simulink model "signalTesting"  (R2024b)
settings: Solver=VariableStepAuto  StartTime=0.0  StopTime=60  RelTol=1e-3
libraries: dspstat3 x12, dspfdesign x6
settings Model: Creator=Mateusz  LastModifiedBy=Mateusz
settings OptimizationCC: ReuseModelBlockBuffer=off
settings RTWCC: GPUComputeCapability=3.5

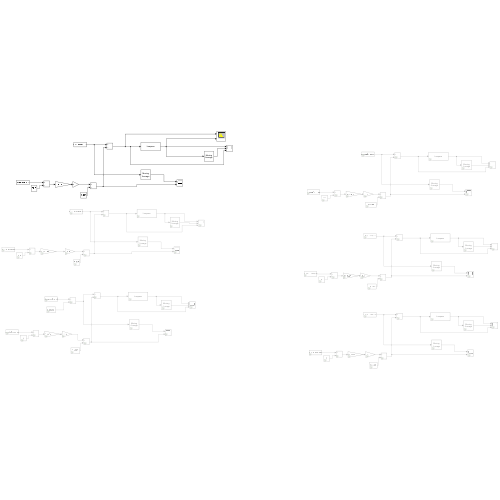
[thumbnail: Simulink's stored preview of the top-level diagram]
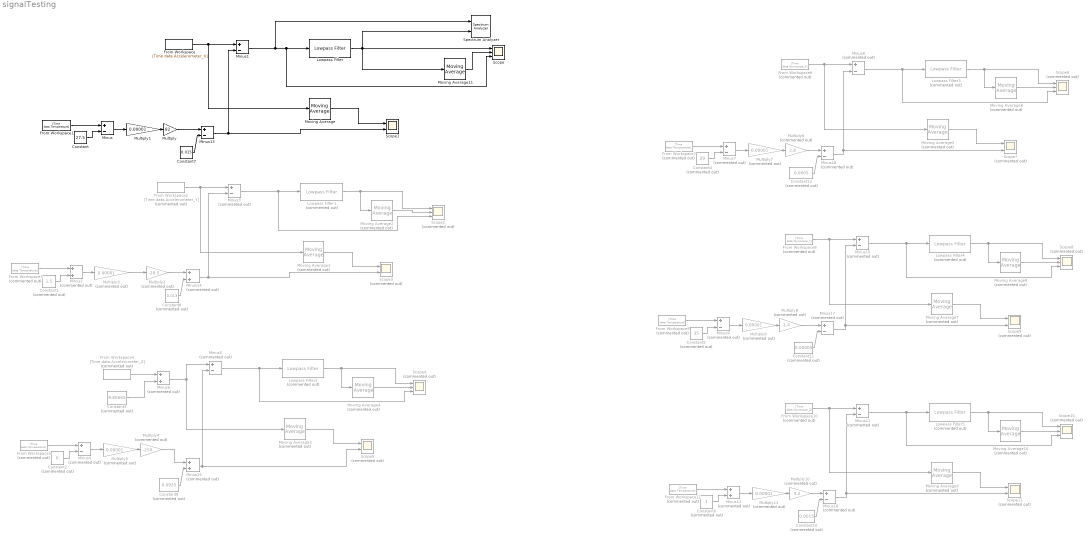
== system signalTesting ==
  Constant : Constant  Value=27.5
  Constant1 : Constant  Commented=on  Value=1.5
  Constant10 : Constant  Commented=on  Value=0.0015
  Constant11 : Constant  Commented=on  Value=0.00005
  Constant12 : Constant  Commented=on  Value=0.0005
  Constant2 : Constant  Commented=on  Value=6
  Constant3 : Constant  Commented=on  Value=9.80665
  Constant4 : Constant  Commented=on  Value=29
  Constant5 : Constant  Commented=on  Value=35
  Constant6 : Constant  Commented=on
  Constant7 : Constant  Value=0.015
  Constant8 : Constant  Commented=on  Value=0.013
  Constant9 : Constant  Commented=on  Value=0.0925
  From Workspace : FromWorkspace  VariableName=[Time data.Accelerometer_X]  SampleTime=0.01
  From Workspace1 : FromWorkspace  VariableName=[Time data.Temperature]  SampleTime=0.01
  From Workspace10 : FromWorkspace  Commented=on  VariableName=[Time data.Gyroscope_Z]  SampleTime=0.01
  From Workspace{3,5,7,9,11} (5 alike) : FromWorkspace  Commented=on  VariableName=[Time data.Temperature]  SampleTime=0.01
  From Workspace2 : FromWorkspace  Commented=on  VariableName=[Time data.Accelerometer_Y]  SampleTime=0.01
  From Workspace4 : FromWorkspace  Commented=on  VariableName=[Time data.Accelerometer_Z]  SampleTime=0.01
  From Workspace6 : FromWorkspace  Commented=on  VariableName=[Time data.Gyroscope_X]  SampleTime=0.01
  From Workspace8 : FromWorkspace  Commented=on  VariableName=[Time data.Gyroscope_Y]  SampleTime=0.01
  Lowpass Filter : dspfdesign/Lowpass Filter  FilterType=FIR  DesignForMinimumOrder=on  FilterOrder=50  PassbandFrequency=0.00001  StopbandFrequency=0.1  PassbandRipple=0.1  StopbandAttenuation=50  SampleRateMode=Use normalized frequency (0 to 1)  SampleRate=44100  SimulateUsing=Interpreted execution  roundingMode=Floor  coeffsDataTypeStr=fixdt(1,16)
  Lowpass Filter{1..5} (5 alike) : dspfdesign/Lowpass Filter  Commented=on  FilterType=FIR  DesignForMinimumOrder=on  FilterOrder=50  PassbandFrequency=0.01  StopbandFrequency=0.2  PassbandRipple=0.01  StopbandAttenuation=60  SampleRateMode=Use normalized frequency (0 to 1)  SampleRate=44100  SimulateUsing=Interpreted execution  roundingMode=Floor  coeffsDataTypeStr=fixdt(1,16)
  Minus : Sum  Inputs=+-
  Minus1 : Sum  Inputs=+-
  Minus{3..5,7..11,16..18} (11 alike) : Sum  Commented=on  Inputs=+-
  Minus{2,6,12,14..15} (5 alike) : Sum  Commented=on
  Minus13 : Sum  Inputs=+-
  Moving Average : dspstat3/Moving Average  Method=Sliding window  ForgettingFactorPort=off  SpecifyWindowLength=on  WindowLength=501  OverlapLength=500  AllowArbitraryInputLength=off  ForgettingFactor=0.9  SimulateUsing=Interpreted execution
  Moving Average{1..10} (10 alike) : dspstat3/Moving Average  Commented=on  Method=Sliding window  ForgettingFactorPort=off  SpecifyWindowLength=on  WindowLength=501  OverlapLength=500  AllowArbitraryInputLength=off  ForgettingFactor=0.9  SimulateUsing=Interpreted execution
  Moving Average11 : dspstat3/Moving Average  Method=Sliding window  ForgettingFactorPort=off  SpecifyWindowLength=on  WindowLength=501  OverlapLength=500  AllowArbitraryInputLength=off  ForgettingFactor=0.9  SimulateUsing=Interpreted execution
  Multiply : Gain  Gain=82
  Multiply1 : Gain  Gain=0.00001
  Multiply10 : Gain  Commented=on  Gain=3.2
  Multiply{3,5,7,9,11} (5 alike) : Gain  Commented=on  Gain=0.00001
  Multiply2 : Gain  Commented=on  Gain=-28.5
  Multiply4 : Gain  Commented=on  Gain=-250
  Multiply6 : Gain  Commented=on  Gain=2.8
  Multiply8 : Gain  Commented=on  Gain=1.4
  Scope : Scope  NumInputPorts=3
  Scope1 : Scope  NumInputPorts=2
  Scope{2,4,6,8,10} (5 alike) : Scope  Commented=on  NumInputPorts=3
  Scope{3,5,7,9,11} (5 alike) : Scope  Commented=on  NumInputPorts=2
  Spectrum Analyzer : SpectrumAnalyzer  NumInputPorts=2  WindowPosition=[-1733.000000,170.000000,1527.000000,785.000000,]  ScopeFrameLocation=window  WindowInvariantSamplesPerUpdate=on  Span=100  StartFrequency=-50  StopFrequency=50  YLimits=[-73.15886504,-26.38842028]
  wires:
  From Workspace/1 -> Moving Average/1, Minus1/1
  Moving Average/1 -> Scope1/1
  Minus/1 -> Multiply1/1
  From Workspace1/1 -> Minus/1
  Constant/1 -> Minus/2
  Multiply1/1 -> Multiply/1
  Minus1/1 -> Spectrum Analyzer/1, Scope/3, Lowpass Filter/1
  Constant1/1 -> Minus2/2
  Minus2/1 -> Multiply3/1
  From Workspace3/1 -> Minus2/1
  Lowpass Filter1/1 -> Moving Average2/1, Scope2/1
  Multiply3/1 -> Multiply2/1
  From Workspace2/1 -> Moving Average1/1, Minus3/1
  Moving Average1/1 -> Scope3/1
  Minus3/1 -> Scope2/3, Lowpass Filter1/1
  Moving Average2/1 -> Scope2/2
  Moving Average4/1 -> Scope4/2
  Moving Average3/1 -> Scope5/1
  Minus5/1 -> Scope4/3, Lowpass Filter2/1
  Multiply5/1 -> Multiply4/1
  Constant2/1 -> Minus4/2
  Lowpass Filter2/1 -> Moving Average4/1, Scope4/1
  Minus4/1 -> Multiply5/1
  From Workspace5/1 -> Minus4/1
  Minus6/1 -> Moving Average3/1, Minus5/1
  From Workspace4/1 -> Minus6/1
  Constant3/1 -> Minus6/2
  Moving Average6/1 -> Scope6/2
  Moving Average5/1 -> Scope7/1
  From Workspace6/1 -> Moving Average5/1, Minus8/1
  Minus8/1 -> Scope6/3, Lowpass Filter3/1
  Multiply7/1 -> Multiply6/1
  Constant4/1 -> Minus7/2
  Lowpass Filter3/1 -> Moving Average6/1, Scope6/1
  Minus7/1 -> Multiply7/1
  From Workspace7/1 -> Minus7/1
  Constant5/1 -> Minus9/2
  Minus10/1 -> Scope8/3, Lowpass Filter4/1
  From Workspace8/1 -> Moving Average7/1, Minus10/1
  Lowpass Filter4/1 -> Moving Average8/1, Scope8/1
  From Workspace9/1 -> Minus9/1
  Multiply9/1 -> Multiply8/1
  Moving Average7/1 -> Scope9/1
  Moving Average8/1 -> Scope8/2
  Minus9/1 -> Multiply9/1
  Multiply11/1 -> Multiply10/1
  Moving Average9/1 -> Scope11/1
  From Workspace10/1 -> Moving Average9/1, Minus11/1
  Moving Average10/1 -> Scope10/2
  Lowpass Filter5/1 -> Moving Average10/1, Scope10/1
  Minus11/1 -> Scope10/3, Lowpass Filter5/1
  Constant6/1 -> Minus12/2
  Minus12/1 -> Multiply11/1
  From Workspace11/1 -> Minus12/1
  Moving Average11/1 -> Scope/2
  Multiply/1 -> Minus13/1
  Minus13/1 -> Minus1/2, Scope1/2
  Constant7/1 -> Minus13/2
  Constant8/1 -> Minus14/2
  Minus14/1 -> Minus3/2, Scope3/2
  Multiply2/1 -> Minus14/1
  Constant9/1 -> Minus15/2
  Multiply4/1 -> Minus15/1
  Minus15/1 -> Scope5/2, Minus5/2
  Constant10/1 -> Minus16/2
  Multiply10/1 -> Minus16/1
  Minus16/1 -> Scope11/2, Minus11/2
  Constant11/1 -> Minus17/2
  Minus17/1 -> Scope9/2, Minus10/2
  Multiply8/1 -> Minus17/1
  Constant12/1 -> Minus18/2
  Multiply6/1 -> Minus18/1
  Minus18/1 -> Scope7/2, Minus8/2
  Lowpass Filter/1 -> Scope/1, Spectrum Analyzer/2, Moving Average11/1
